simulink model "lab06_Introduction_to_Simulink"  (R2022b)
settings: Solver=FixedStepAuto  StartTime=0.0  StopTime=10.0  FixedStep=1e-3  RelTol=1e-3
settings Model: Creator=MAAM  LastModifiedBy=MAAM

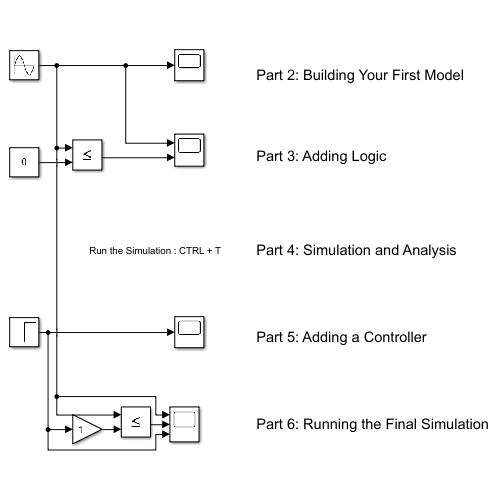
[thumbnail: Simulink's stored preview of the top-level diagram]
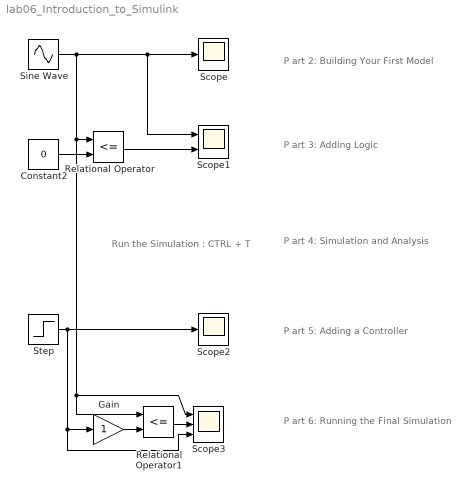
== system lab06_Introduction_to_Simulink ==
  note: Run the Simulation : CTRL + T
  note: P art 6: Running the Final Simulation
  note: P art 5: Adding a Controller
  note: P art 4: Simulation and Analysis
  note: P art 3: Adding Logic
  note: P art 2: Building Your First Model
  Constant2 : Constant  Value=0
  Gain : Gain
  Relational Operator : RelationalOperator  Operator=<=  OutDataTypeStr=boolean  RndMeth=Simplest  InputSameDT=off
  Relational Operator1 : RelationalOperator  Operator=<=  OutDataTypeStr=boolean  RndMeth=Simplest  InputSameDT=off
  Scope : Scope
  Scope1 : Scope  NumInputPorts=2
  Scope2 : Scope
  Scope3 : Scope  NumInputPorts=3
  Sine Wave : Sin  Frequency=2*pi*1  SampleTime=0
  Step : Step  Time=2  SampleTime=0
  wires:
  Sine Wave/1 -> Scope3/1, Relational Operator1/1, Relational Operator/1, Scope1/1, Scope/1
  Constant2/1 -> Relational Operator/2
  Relational Operator/1 -> Scope1/2
  Step/1 -> Scope2/1, Scope3/3, Gain/1
  Gain/1 -> Relational Operator1/2
  Relational Operator1/1 -> Scope3/2
